simulink library "Pump_basic"  (R2018b)
settings: Solver=ode45  StartTime=0.0  StopTime=10.0  RelTol=1e-3  EnableMultiTasking=on
undefined symbols (not defined in the file): MassFlow, Temperature, Water
libraries: carnot x1
settings Model: Creator=lena.frank  LastModifiedBy=P41573
settings DataIOCC: LimitDataPoints=on  SaveFormat=Array  SignalLoggingSaveFormat=ModelDataLogs
settings OptimizationCC: ExpressionDepthLimit=2147483647  LifeSpan=inf
settings DebuggingCC: UnderspecifiedInitializationDetection=Classic  MergeDetectMultiDrivingBlocksExec=none  SolverPrmCheckMsg=warning  FcnCallInpInsideContextMsg=warning  StateNameClashWarn=warning  SFUnexpectedBacktrackingDiag=warning  SFNoUnconditionalDefaultTransitionDiag=warning  SFExecutionAtInitializationDiag=none
settings HardwareCC: ProdBitPerPointer=32  ProdBitPerSizeT=32  ProdBitPerPtrDiffT=32  ProdLargestAtomicFloat=None  ProdIntDivRoundTo=Undefined  ProdEndianess=Unspecified  ProdWordSize=32  ProdHWDeviceType=32-bit Generic
settings ModelReferenceCC: PropagateSignalLabelsOutOfModel=off
settings SFSimCC: SimUseLocalCustomCode=off
settings RTWCC: RTWUseLocalCustomCode=off
settings CodeAppCC: StateflowObjectComments=on
settings GRTTargetCC: TargetLangStandard=C89/C90 (ANSI)  GeneratePreprocessorConditionals=Disable all  CombineOutputUpdateFcns=off  GRTInterface=on
settings ConfigComp: CovMetricSettings=dw  CovHtmlReporting=on  CovSaveCumulativeToWorkspaceVar=on  CovSaveSingleToWorkspaceVar=on  CovExternalEMLEnable=off

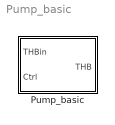
== system Pump_basic ==
  Pump_basic : Subsystem  mask(basic Pump){mdotmax=0.1, fluid_id=Water, mix=0, mix2=0, mix3=0, p0=3e5, dia=0.02, ID=No Pressure Drop, hgt=0}
      mask prompts: mdotmax "massflow rate [kg/s]"; fluid_id "fluid"; mix "percentage of fluid mix [0..1]"; mix2 "fluid mixture 2 [0..1]"; mix3 "fluid mixture 3 [0..1]"; p0 "system pressure [Pa]"; dia "diameter at in- and outlet [m]"; ID "ID (pressure drop calculation mode)"; hgt "static height in m (positive value above ground)"
      mask help:
      | Set constant massflow rate according to the control signal.
      | ID for pressure drop calculation:
      |     1    .. 9999 No Pressure Drop
      |     10001..19999 Pressure Drop from Massflow
      |     20001..inf   Full Pressure Drop with Static Height
      mask init:
      | mix = min(1, max(0, mix));
      | dia = max(0.001, dia);
      mask Help: web(fullfile(path_carnot('help'),'Pump_basic.html'),'-helpbrowser')
      mask TypeOptions mdotmax: mdot/Gain
      mask TypeOptions fluid_id: basic_THB/fluid
      mask TypeOptions mix: basic_THB/mix
      mask TypeOptions mix2: basic_THB/mix2
      mask TypeOptions mix3: basic_THB/mix3
      mask TypeOptions p0: basic_THB/p
      mask TypeOptions dia: basic_THB/dia
      mask TypeOptions ID: basic_THB/ID
      mask TypeOptions hgt: basic_THB/hgt
      mask Display:
      | plot(0,0,100,100, ...
      |     [40,70,40,30,30,40,60,70,70,60,40],[70,50,30,40,60,70,70,60,40,30,30])

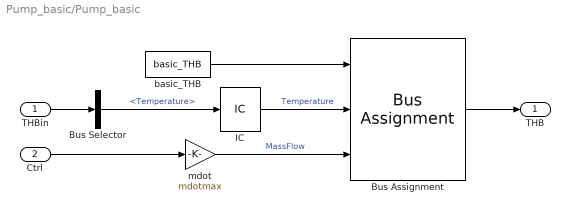
== system Pump_basic/Pump_basic ==
  THBin : Inport
  Ctrl : Inport  Port=2
  Bus Assignment : BusAssignment  AssignedSignals=Temperature,MassFlow
  Bus Selector : BusSelector  OutputSignals=Temperature
  IC : InitialCondition  Value=20
  basic_THB : carnot/Basic/Hydraulics/basic_THB  t=20  mdot=0  p=p0  ID=No Pressure Drop  fluid=Water  mix=mix  mix2=mix2  mix3=mix3  dia=dia  hgt=hgt
      settings: SourceProductName=Carnot
  mdot : Gain  Gain=mdotmax  SaturateOnIntegerOverflow=on  OutDataTypeStr=Inherit: Same as input  ParamDataTypeStr=Inherit: Same as input
  THB : Outport
  wires:
  Bus Assignment/1 -> THB/1
  basic_THB/1 -> Bus Assignment/1
  Bus Selector/1 -> IC/1  "<Temperature>"
  THBin/1 -> Bus Selector/1
  Ctrl/1 -> mdot/1
  mdot/1 -> Bus Assignment/3  "MassFlow"
  IC/1 -> Bus Assignment/2  "Temperature"
